simulink model "fuzzyTradPid"  (R2022a)
settings: Solver=VariableStepAuto  StartTime=0.0  StopTime=0.1  RelTol=1e-3
libraries: fuzblock x1
settings Model: Creator=FLKU  LastModifiedBy=FLKU

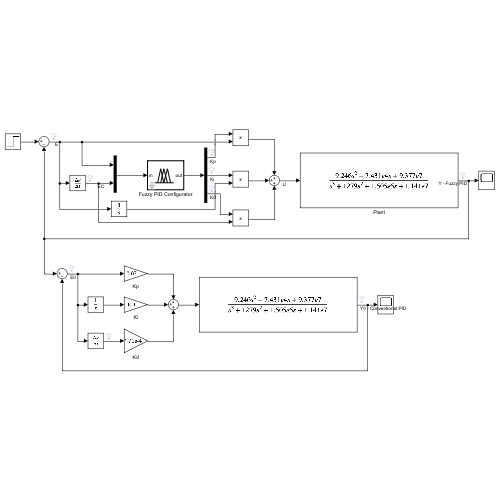
[thumbnail: Simulink's stored preview of the top-level diagram]
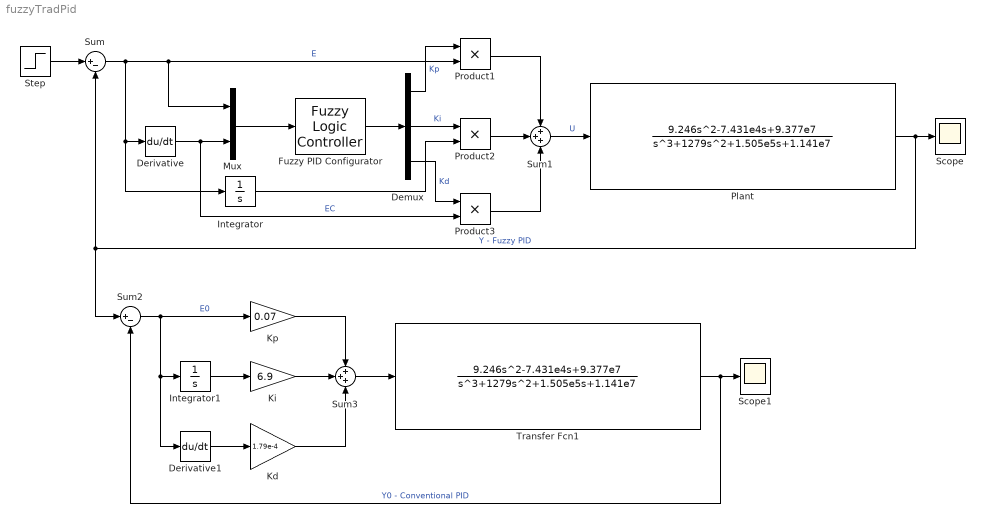
== system fuzzyTradPid ==
  Demux : Demux  Outputs=3
  Derivative : Derivative
  Derivative1 : Derivative
  Fuzzy PID Configurator : fuzblock/Fuzzy Logic  Controller  FIS=fistrad  OutputSampleNumber=101  DataType=double  FuzzifiedInputs=off  RuleFiringStrengths=off  RuleOutputs=off  AggregatedOutputs=off  SimulateUsing=Interpreted execution  OutOfRangeInputValueMessage=warning  NoRuleFiredMessage=error  EmptyOutputFuzzySetMessage=error
  Integrator : Integrator
  Integrator1 : Integrator
  Kd : Gain  Gain=1.79e-4
  Ki : Gain  Gain=6.9
  Kp : Gain  Gain=0.07
  Mux : Mux  Inputs=2
  Plant : TransferFcn  Numerator=[9.246 -7.431e4 9.377e7]  Denominator=[1 1279 1.505e5 1.141e7]  ContinuousStateAttributes='position'
  Product1 : Product
  Product2 : Product
  Product3 : Product
  Scope : Scope
  Scope1 : Scope
  Step : Step  Time=0  SampleTime=0
  Sum : Sum  Inputs=|+-
  Sum1 : Sum  Inputs=+++
  Sum2 : Sum  Inputs=|+-
  Sum3 : Sum  Inputs=+++
  Transfer Fcn1 : TransferFcn  Numerator=[9.246 -7.431e4 9.377e7]  Denominator=[1 1279 1.505e5 1.141e7]  ContinuousStateAttributes='position'
  wires:
  Step/1 -> Sum/1
  Integrator/1 -> Product2/2
  Mux/1 -> Fuzzy PID Configurator/1
  Product1/1 -> Sum1/1
  Sum1/1 -> Plant/1  "U"
  Product3/1 -> Sum1/3
  Fuzzy PID Configurator/1 -> Demux/1
  Sum/1 -> Integrator/1, Derivative/1, Mux/1, Product1/2  "E"
  Demux/1 -> Product1/1  "Kp"
  Demux/2 -> Product2/1  "Ki"
  Demux/3 -> Product3/1  "Kd"
  Derivative/1 -> Mux/2, Product3/2  "EC"
  Product2/1 -> Sum1/2
  Plant/1 -> Sum/2, Sum2/1, Scope/1  "Y - Fuzzy PID"
  Sum2/1 -> Derivative1/1, Integrator1/1, Kp/1  "E0"
  Kp/1 -> Sum3/1
  Ki/1 -> Sum3/2
  Derivative1/1 -> Kd/1
  Transfer Fcn1/1 -> Sum2/2, Scope1/1  "Y0 - Conventional PID"
  Sum3/1 -> Transfer Fcn1/1
  Integrator1/1 -> Ki/1
  Kd/1 -> Sum3/3
